simulink model "sat_v4"  (R2020a)
settings: Solver=FixedStepAuto  StartTime=0.0  StopTime=10.0  RelTol=1e-3  EnableMultiTasking=on
PreLoadFcn:
  | step_size = 0.001;
InitFcn:
  | step_size = 0.001;
StartFcn:
  | step_size = 0.001;
libraries: arduinolib x14, simulink x1
settings Model: SILPILModeSetting=veronly  ExtModeTrigDuration=2  Creator=hend_aafia  LastModifiedBy=hend_aafia
settings SolverCC: AutoInsertRateTranBlk=on
settings OptimizationCC: EnhancedBackFolding=on  PassReuseOutputArgsAs=Individual arguments  ZeroExternalMemoryAtStartup=off  ZeroInternalMemoryAtStartup=off  MaxStackSize=64  OptimizeBlockOrder=speed  DifferentSizesBufferReuse=on  OptimizationCustomize=off  EfficientTunableParamExpr=on
settings DebuggingCC: ParameterTunabilityLossMsg=error
settings HardwareCC: ProdBitPerInt=16  ProdBitPerPointer=16  ProdBitPerSizeT=16  ProdBitPerPtrDiffT=16  ProdLargestAtomicFloat=None  ProdWordSize=8  ProdHWDeviceType=Atmel->AVR
settings SFSimCC: MATLABDynamicMemAlloc=off
settings RTWCC: SystemTargetFile=ert.tlc  HardwareBoard=Arduino Mega 2560  TLCOptions=-aInlineSetEventsForThisBaseRateFcn=TLC_FALSE -aSuppressMultiTaskScheduler=TLC_FALSE -aRateBasedStepFcn=1  TemplateMakefile=ert_default_tmf  Toolchain=Arduino AVR  BuildConfiguration=Faster Runs
settings CodeAppCC: ForceParamTrailComments=on  IgnoreCustomStorageClasses=off  OperatorAnnotations=on  SimulinkDataObjDesc=on  SFDataObjDesc=on  InsertBlockDesc=on
settings ERTTargetCC: SupportContinuousTime=on  SupportVariableSizeSignals=on  ExtModeStaticAllocSize=2048

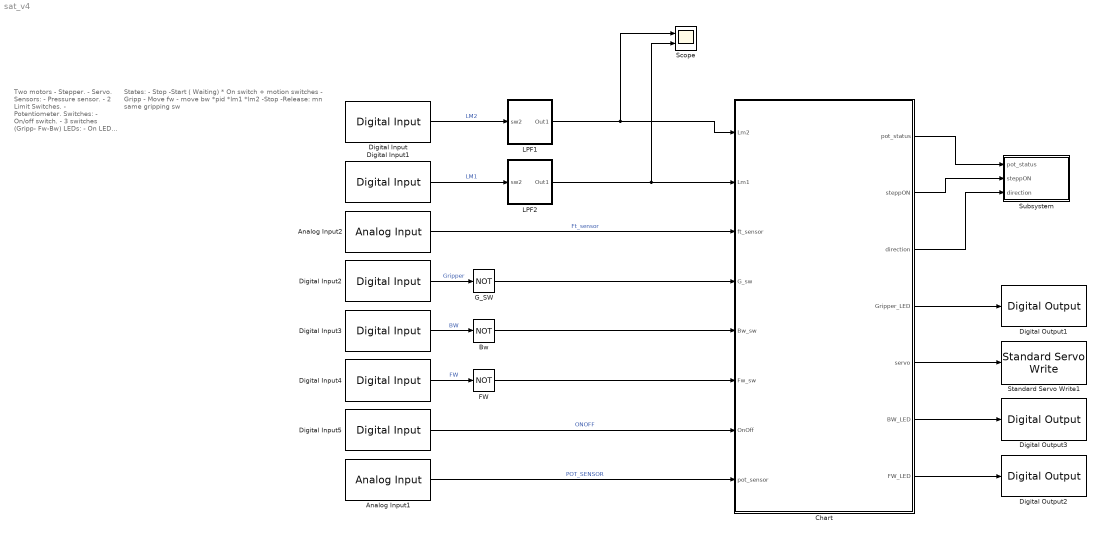
== system sat_v4 ==
  note: Two motors
      | - Stepper.
      | - Servo.
      |
      | Sensors:
      | - Pressure sensor.
      | - 2 Limit Switches.
      | - Potentiometer.
      |
      | Switches:
      | - On/off switch.
      | - 3 switches (Gripp- Fw-Bw)
      |
      | LEDs:
      | - On LED
      | - Gripper LED
      |
      | - Gripper LED
      | - Fw LED
      | - Bw LED
  note: States:
      | - Stop
      | -Start ( Waiting)
      |
      | * On switch + motion switches
      |
      | - Gripp - Move fw - move bw
      |
      | *pid *lm1 *lm2
      |
      | -Stop
      | -Release:
      | mn same gripping sw
  Analog Input1 : arduinolib/Analog Input  pinNumber=1  ReadResultsOnly=off  ConversionTriggerSource=Software  ExternalTriggerType=uint32( 0 )  OutputDataType=uint16  EnableConversionCompleteNotify=off  EnableOuputStatus=off  SampleTime=-1  blockPlatform=arduino
  Analog Input2 : arduinolib/Analog Input  pinNumber=0  ReadResultsOnly=off  ConversionTriggerSource=Software  ExternalTriggerType=uint32( 0 )  OutputDataType=uint16  EnableConversionCompleteNotify=off  EnableOuputStatus=off  SampleTime=-1  blockPlatform=arduino
  Bw : Logic  Operator=NOT  IconShape=distinctive  AllPortsSameDT=off  OutDataTypeStr=boolean
  Chart : Stateflow chart  TreatAsAtomicUnit=on
  Digital Input : arduinolib/Digital Input  pinNumber=4  Direction=input  SampleTime=step_size  blockPlatform=arduino
  Digital Input1 : arduinolib/Digital Input  pinNumber=5  Direction=input  SampleTime=step_size  blockPlatform=arduino
  Digital Input2 : arduinolib/Digital Input  pinNumber=6  Direction=input  SampleTime=step_size  blockPlatform=arduino
  Digital Input3 : arduinolib/Digital Input  pinNumber=10  Direction=input  SampleTime=step_size  blockPlatform=arduino
  Digital Input4 : arduinolib/Digital Input  pinNumber=7  Direction=input  SampleTime=step_size  blockPlatform=arduino
  Digital Input5 : arduinolib/Digital Input  pinNumber=11  Direction=input  SampleTime=step_size  blockPlatform=arduino
  Digital Output1 : arduinolib/Digital Output  pinNumber=12  Direction=output  blockPlatform=arduino
  Digital Output2 : arduinolib/Digital Output  pinNumber=13  Direction=output  blockPlatform=arduino
  Digital Output3 : arduinolib/Digital Output  pinNumber=8  Direction=output  blockPlatform=arduino
  FW : Logic  Operator=NOT  IconShape=distinctive  AllPortsSameDT=off  OutDataTypeStr=boolean
  G_SW : Logic  Operator=NOT  IconShape=distinctive  AllPortsSameDT=off  OutDataTypeStr=boolean
  LPF1 : Subsystem
  LPF2 : Subsystem
  Scope : Scope  NumInputPorts=2
  Standard Servo Write1 : arduinolib/Standard Servo Write  pinNumber=9  ServoIndex=0  blockPlatform=arduino
  Subsystem : Subsystem
  wires:
  Chart/7(FW_LED) -> Digital Output2/1
  Chart/3(direction) -> Subsystem/3(direction)
  FW/1 -> Chart/6(Fw_sw)
  Chart/2(steppON) -> Subsystem/2("steppON ")
  Digital Input4/1 -> FW/1  "FW"
  Analog Input1/1 -> Chart/8(pot_sensor)  "POT_SENSOR"
  Digital Input3/1 -> Bw/1  "BW"
  Digital Input/1 -> LPF1/1(sw2)  "LM2"
  Digital Input1/1 -> LPF2/1(sw2)  "LM1"
  Digital Input5/1 -> Chart/7(OnOff)  "ONOFF"
  Bw/1 -> Chart/5(Bw_sw)
  Chart/6(BW_LED) -> Digital Output3/1
  Chart/1(pot_status) -> Subsystem/1(pot_status)
  Analog Input2/1 -> Chart/3(ft_sensor)  "Ft_sensor"
  G_SW/1 -> Chart/4(G_sw)
  Digital Input2/1 -> G_SW/1  "Gripper"
  Chart/4(Gripper_LED) -> Digital Output1/1
  Chart/5(servo) -> Standard Servo Write1/1
  LPF1/1(Out1) -> Scope/1, Chart/1(Lm2)
  LPF2/1(Out1) -> Scope/2, Chart/2(Lm1)

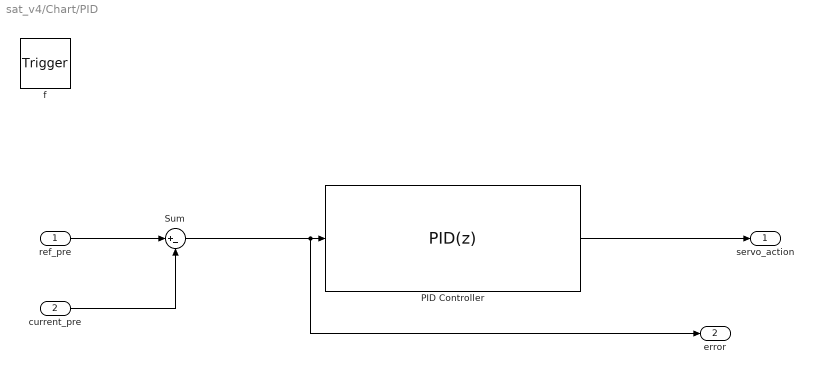
== system sat_v4/Chart/PID ==
  ref_pre : Inport  OutMin=-1000  OutMax=1000  OutDataTypeStr=double  Unit=N/(m^2)  PortDimensions=1
  current_pre : Inport  Port=2  OutDataTypeStr=uint16  Unit=N/(m^2)  PortDimensions=1
  f : TriggerPort  TriggerType=function-call  VariantControl=(inherit)
      settings: CopyFcn=Stateflow.SLINSF.SimulinkMan.removeBlockPreDeleteFcn  PreDeleteFcn=Stateflow.SLINSF.SimulinkMan.unsafePredeleteFcn
  PID Controller : simulink/Continuous/PID Controller  Controller=PID  Form=Parallel  TimeDomain=Discrete-time  UseExternalTs=off  SampleTime=-1  IntegratorMethod=Forward Euler  FilterMethod=Forward Euler  ControllerParametersSource=internal  P=0.001  I=0  D=0.005  UseFilter=on  N=100  TunerSelectOption=Transfer Function Based (PID Tuner App)  InitialConditionSource=internal  InitialConditionForIntegrator=0  InitialConditionForFilter=0  DifferentiatorICPrevScaledInput=0  ExternalReset=none  TrackingMode=off  Kt=1  LimitOutput=off  UpperSaturationLimit=inf  LowerSaturationLimit=-inf  LinearizeAsGain=on  AntiWindupMode=none  Kb=1  PGainOutDataTypeStr=double  PProdOutDataTypeStr=double  POutMin=[]  POutMax=[]  IOutMin=[]  IOutMax=[]  DOutMin=[]  DOutMax=[]  NOutMin=[]  NOutMax=[]  SumOutMin=[]  SumOutMax=[]  SaturationOutMin=[]  SaturationOutMax=[]  PParamMin=[]  PParamMax=[]  IParamMin=[]  IParamMax=[]  DParamMin=[]  DParamMax=[]  NParamMin=[]  NParamMax=[]  KbParamMin=[]  KbParamMax=[]  KtParamMin=[]  KtParamMax=[]  KbOutMin=[]  KbOutMax=[]  KtOutMin=[]  KtOutMax=[]  IntegratorOutMin=[]  IntegratorOutMax=[]  FilterOutMin=[]  FilterOutMax=[]  SumI1OutMin=[]  SumI1OutMax=[]  SumI2OutMin=[]  SumI2OutMax=[]  SumI3OutMin=[]  SumI3OutMax=[]  SumI4OutMin=[]  SumI4OutMax=[]  SumDOutMin=[]  SumDOutMax=[]  DifferentiatorOutMin=[]  DifferentiatorOutMax=[]  FilterDiffOutCoefMin=[]  FilterDiffOutCoefMax=[]  ReciprocalOutMin=[]  ReciprocalOutMax=[]  SumDenOutMin=[]  SumDenOutMax=[]  SumNumOutMin=[]  SumNumOutMax=[]  DivideOutMin=[]  DivideOutMax=[]  UdiffTsProdOutMin=[]  UdiffTsProdOutMax=[]  NTsProdOutMin=[]  NTsProdOutMax=[]  UintegralTsProdOutMin=[]  UintegralTsProdOutMax=[]  UngainTsProdOutMin=[]  UngainTsProdOutMax=[]  IntegratorContinuousStateAttributes=''  IntegratorStateMustResolveToSignalObject=off  IntegratorRTWStateStorageClass=Auto  FilterContinuousStateAttributes=''  FilterStateMustResolveToSignalObject=off  FilterRTWStateStorageClass=Auto  ParallelPVariant=InternalParameters  IdealPVariant=Disabled  IVariant=InternalParameters  DVariant=InternalParameters  IntegratorVariant=Discrete  SatVariant=Disabled  AWVariant=Passthrough  PCopyVariant=Disabled  TRVariant=Disabled  FdbkBlocksVariant=Forward  IdealPFdbkVariant=Disabled  SatFdbkVariant=Disabled  DerivativeFilterVariant=ForwardEulerFilter  NVariant=InternalParameters  NCopyVariant=Disabled  FilterICVariant=InternalICsFilter  IntegratorICVariant=InternalICs  ExternalResetVariant=Disabled  TRSumVariant=Passthrough  SumFdbkVariant=Disabled  SumVariant=Sum_PID  TsampFilterVariant=InternalTs  TsampNgainVariant=Passthrough  TsampIntegralVariant=Passthrough
  Sum : Sum  Inputs=|+-
  servo_action : Outport
  error : Outport  Port=2
  wires:
  ref_pre/1 -> Sum/1
  PID Controller/1 -> servo_action/1
  current_pre/1 -> Sum/2
  Sum/1 -> error/1, PID Controller/1

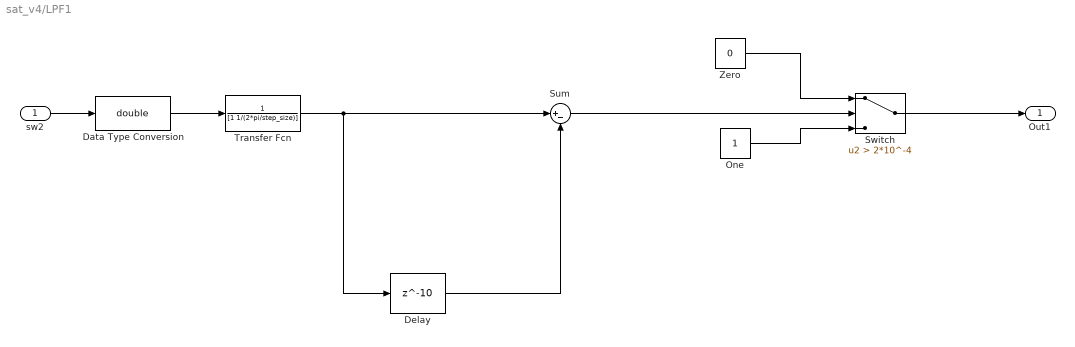
== system sat_v4/LPF1 ==
  sw2 : Inport
  Data Type Conversion : DataTypeConversion  OutDataTypeStr=double
  Delay : Delay  DelayLength=10  InputProcessing=Columns as channels (frame based)
  One : Constant  OutDataTypeStr=Inherit: Inherit via back propagation
  Sum : Sum  Inputs=|+-
  Switch : Switch  Criteria=u2 > Threshold  Threshold=2*10^-4
  Transfer Fcn : TransferFcn  Denominator=[1 1/(2*pi/step_size)]
  Zero : Constant  Value=0  OutDataTypeStr=Inherit: Inherit via back propagation
  Out1 : Outport
  wires:
  Delay/1 -> Sum/2
  One/1 -> Switch/3
  Zero/1 -> Switch/1
  Data Type Conversion/1 -> Transfer Fcn/1
  sw2/1 -> Data Type Conversion/1
  Switch/1 -> Out1/1
  Sum/1 -> Switch/2
  Transfer Fcn/1 -> Sum/1, Delay/1

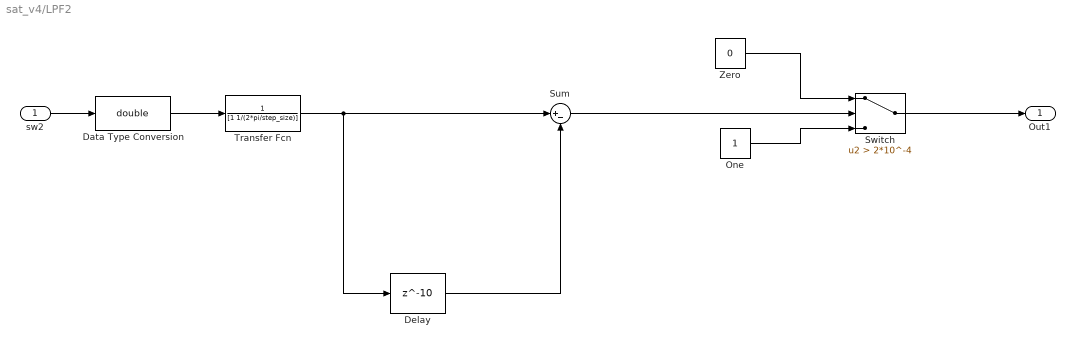
== system sat_v4/LPF2 ==
  sw2 : Inport
  Data Type Conversion : DataTypeConversion  OutDataTypeStr=double
  Delay : Delay  DelayLength=10  InputProcessing=Columns as channels (frame based)
  One : Constant  OutDataTypeStr=Inherit: Inherit via back propagation
  Sum : Sum  Inputs=|+-
  Switch : Switch  Criteria=u2 > Threshold  Threshold=2*10^-4
  Transfer Fcn : TransferFcn  Denominator=[1 1/(2*pi/step_size)]
  Zero : Constant  Value=0  OutDataTypeStr=Inherit: Inherit via back propagation
  Out1 : Outport
  wires:
  Transfer Fcn/1 -> Delay/1, Sum/1
  Sum/1 -> Switch/2
  Switch/1 -> Out1/1
  sw2/1 -> Data Type Conversion/1
  Data Type Conversion/1 -> Transfer Fcn/1
  Zero/1 -> Switch/1
  One/1 -> Switch/3
  Delay/1 -> Sum/2

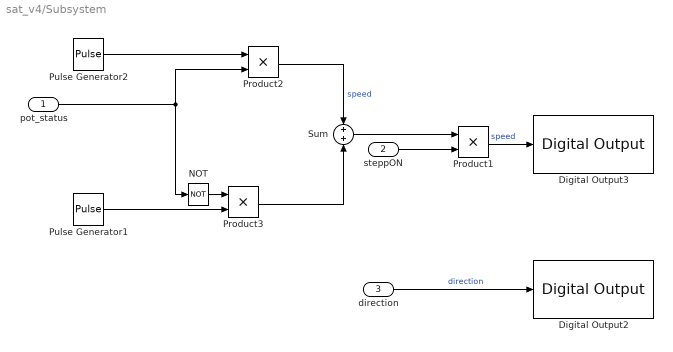
== system sat_v4/Subsystem ==
  pot_status : Inport
  "steppON " : Inport  Port=2
  direction : Inport  Port=3
  Digital Output2 : arduinolib/Digital Output  pinNumber=2  Direction=output  blockPlatform=arduino
  Digital Output3 : arduinolib/Digital Output  pinNumber=3  Direction=output  blockPlatform=arduino
  NOT : Logic  Operator=NOT  IconShape=distinctive  AllPortsSameDT=off  OutDataTypeStr=boolean
  Product1 : Product
  Product2 : Product
  Product3 : Product
  Pulse Generator1 : DiscretePulseGenerator  PulseType=Time based  Period=step_size*10  PulseWidth=50
  Pulse Generator2 : DiscretePulseGenerator  PulseType=Time based  Period=step_size  PulseWidth=50
  Sum : Sum
  wires:
  Product3/1 -> Sum/2
  Product1/1 -> Digital Output3/1  "speed"
  Pulse Generator2/1 -> Product2/1
  "steppON "/1 -> Product1/2
  pot_status/1 -> NOT/1, Product2/2
  direction/1 -> Digital Output2/1  "direction"
  NOT/1 -> Product3/1
  Pulse Generator1/1 -> Product3/2
  Product2/1 -> Sum/1  "speed"
  Sum/1 -> Product1/1

== stateflow chart sat_v4/Chart ==
  state Stop
    en:
    servo = 160;
  state [servo_action,error] = PID(ref_pre,current_pre) [function]
  state Start
    en:
    PID_done =0;
    steppON = 0;
    FW_LED =0;
    BW_LED =0;
    servo = 160;
    Gripper_LED = 0;
    if pot_sensor > 500
    pot_status = 0;
    else
    pot_status =1;
    end
  state FW
    during:
    FW_LED  = 1;
    direction = 1;
    steppON = 1;
  state Gripper
    en:
    Gripper_LED = 1;
    if ft_sensor <200
    [ser, error]=PID(400,ft_sensor);
    servo = 160 - ser;
    if (ft_sensor > 400 || ft_sensor == 400 || abs(400 - ft_sensor) <5)
    PID_done = 1;
    end
    end
  state BW
    during:
    BW_LED  = 1;
    direction = 0;
    steppON = 1;
  (default) -> Stop
  Gripper -> Stop [order 2] : [OnOff == 0]
  BW -> Stop [order 1] : [OnOff == 0]
  FW -> Stop [order 1] : [OnOff ==0]
  Start -> Stop [order 1] : [OnOff==0]
  Stop -> Start : [OnOff==1]
  Start -> FW [order 2] : [Fw_sw ==1 && Lm2 == 0 ]
  Start -> Gripper [order 3] : [(G_sw == 1)]
  FW -> Start [order 2] : [Lm2 == 1|| Fw_sw == 0]
  Gripper -> Start [order 1] : [(G_sw == 0)]
  BW -> Start [order 2] : [Lm1==1 || Bw_sw == 0]
  Start -> BW [order 4] : [Bw_sw == 1&& Lm1 == 0]
  data: ref_pre function_input double size=1; current_pre function_input uint16 size=1; servo_action function_output; error function_output; Lm2 input; Lm1 input; ft_sensor input; G_sw input; Bw_sw input; Fw_sw input; OnOff input; pot_status output; steppON output; direction output; PID_done local; Gripper_LED output; pos local; pot_sensor input; ser local; servo output; BW_LED output; FW_LED output; error local; is_gripped local
